simulink model "worm_model"  (R2024a)
settings: Solver=VariableStepAuto  StartTime=0.0  StopTime=24  RelTol=1e-3
model workspace (MAT data in the model file):
  worm_model_spesession : sldodialogs.data.SessionData (value not decoded)
values from neighbouring files (symbols this model uses):
  Bm = 0.00282489539624    [ws_pe_210rpm.mat]
  Jm = 0.00680365875829    [ws_pe_210rpm.mat]
  Kb = 0.568585930411    [ws_pe_210rpm.mat]
  Kt = 1.27385648833    [ws_pe_210rpm.mat]
  L = 0.00045    [ws_pe_210rpm.mat]
  N = 1    [ws_pe_210rpm.mat]
  Ra = 9.86087769042    [ws_pe_210rpm.mat]
settings Model: Creator=iT  LastModifiedBy=Mostafa
settings DataIOCC: ExternalInput=tpd6d99da0_0f5e_435b_8ba7_745dcdb194d8(1)  LoadExternalInput=on  OutputOption=AdditionalOutputTimes  OutputTimes=SDO_OutputTimes  ReturnWorkspaceOutputsName=SDOSimTest_Log
settings RTWCC: GPUComputeCapability=3.5

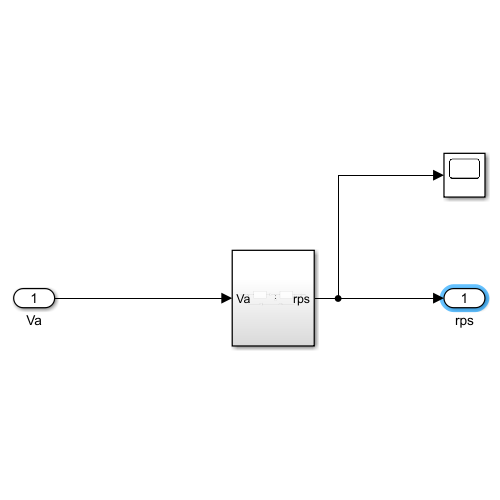
[thumbnail: Simulink's stored preview of the top-level diagram]
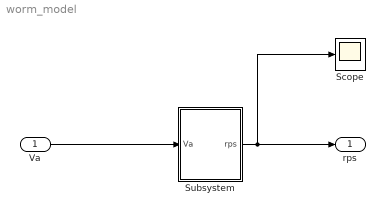
== system worm_model ==
  Va : Inport
  Scope : Scope
  Subsystem : Subsystem
  rps : Outport
  wires:
  Subsystem/1(rps) -> Scope/1, rps/1
  Va/1 -> Subsystem/1(Va)

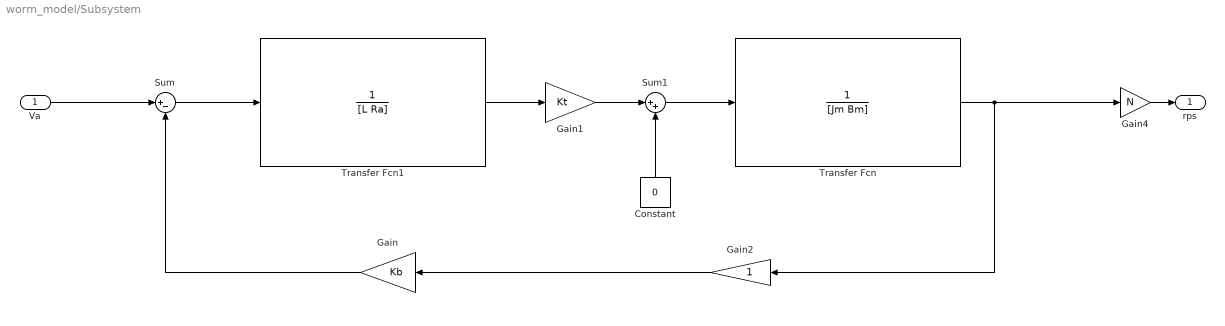
== system worm_model/Subsystem ==
  Va : Inport
  Constant : Constant  Value=0
  Gain : Gain  Gain=Kb
  Gain1 : Gain  Gain=Kt
  Gain2 : Gain
  Gain4 : Gain  Gain=N
  Sum : Sum  Inputs=|+-
  Sum1 : Sum  Inputs=|++
  Transfer Fcn : TransferFcn  Denominator=[Jm Bm]
  Transfer Fcn1 : TransferFcn  Denominator=[L Ra]
  rps : Outport
  wires:
  Sum/1 -> Transfer Fcn1/1
  Gain/1 -> Sum/2
  Constant/1 -> Sum1/2
  Transfer Fcn1/1 -> Gain1/1
  Gain1/1 -> Sum1/1
  Sum1/1 -> Transfer Fcn/1
  Gain2/1 -> Gain/1
  Va/1 -> Sum/1
  Transfer Fcn/1 -> Gain4/1, Gain2/1
  Gain4/1 -> rps/1
